simulink library "PowerFlowLib2013a"  (Simulink 8.1)
settings: Solver=ode45  StartTime=0.0  StopTime=10.0  RelTol=1e-3
undefined symbols (not defined in the file or in its folder): AirProp, C, F1, Fanmap, Fld1, Fld2, fueltankdata, HydProp, HydraulicLoad, IBFD_exc, L, LoadFluidProps, magnitude, MSSN, n_alghts, PumpProp, pwr_alghts, R_fd_exc, Rcore, Ts, VBFD_exc
libraries: PowerFlowLib x32, simulink x14, powerlib_extras x2, dspstat3 x2
(part 1 of 11)
settings Model: Creator=mwillms4  LastModifiedBy=srikanthan

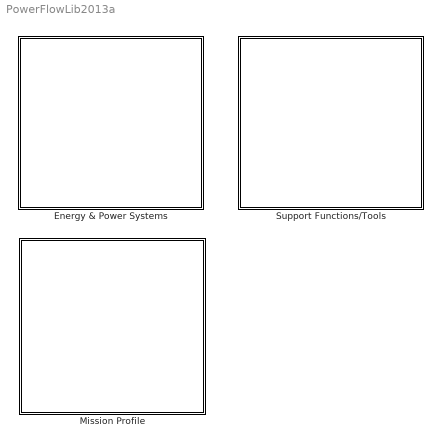
== system PowerFlowLib2013a ==
  Energy & Power Systems : Subsystem
      mask Display: color('white')
  Mission Profile : Subsystem
      mask Display: color('white')
  Support Functions/Tools : Subsystem
      mask Display: color('white')

== system PowerFlowLib2013a/Energy & Power Systems ==
  Additional Systems : Subsystem
  Electrical : Subsystem
  Hydraulic : Subsystem
  Thermal : Subsystem

== system PowerFlowLib2013a/Mission Profile ==
  Mission Profile : Subsystem  mask(MISSION PROFILE SELECT){mssn_check=off, mssn_prof=MSSN, del_P=0, del_T=0, del_rho=0, pres_msl=101.3, temp_msl=15, dens_msl=1.229}
      mask prompts: mssn_check "Define new mission?"; mssn_prof "Mission Profile Variable (from workspace)"; del_P "Pres. deviation from standard atmospheric conditions [kPa]"; del_T "Temp. deviation from standard atmospheric conditions [°C]"; del_rho "Density Deviation from standard"; pres_msl "MSL Pressure [kPa]"; temp_msl "MSL Temperature [°C]"; dens_msl "MSL Density [kg/m³]"
      mask help:
      | Select the MATLAB workspace variable that contains mission specifications. This variable should be created with the automated code included with the PowerFlow toolset.
      |
      | Also specify deviations from standard atmospheric conditions.
      mask init:
      | %{
      | h      = get_param(gcb,'handle');   % Get block handle
      | blk    = gcb; 
      | hblock = get(h);     % Parse out handles structure 
      | 
      | % altitude - row 2 of mission profile
      | set_param([blk,'/ALT'],'Table',[hblock.mssn_prof,'(2,:)'])
      | % mach number - row 22 of mission profile
      | set_param([blk,'/MACH'],'Table',[hblock.mssn_prof,'(22,:)'])
      | % mission phase - row 21 of mission profile
      | set_param([blk,'/MSSN Phase'],'Table',[hblock.mssn_prof,'(21,:)'])
      | % engine 1 on/off - row 6 of mission profile
      | set_param([blk,'/Engine 1'],'Table',[hblock.mssn_prof,'(6,:)'])
      | % engine 2 on/off - row 10 of mission profile
      | set_param([blk,'/Engine 2'],'Table',[hblock.mssn_prof,'(10,:)'])
      | % APU on/off - row 3 of mission profile
      | set_param([blk,'/APU'],'Table',[hblock.mssn_prof,'(3,:)'])
      | % taxi lights - row 16 of mission profile
      | set_param([blk,'/Taxi Lights'],'Table',[hblock.mssn_prof,'(16,:)'])
      | % landing lights - row 17 of mission profile
      | set_param([blk,'/Landing Lights'],'Table',[hblock.mssn_prof,'(17,:)'])
      | % pressurization - row 20 of mission profile
      | set_param([blk,'/Pressurization'],'Table',[hblock.mssn_prof,'(20,:)'])
      | % flaps - row 19 of mission profile
      | set_param([blk,'/Flaps'],'Table',[hblock.mssn_prof,'(19,:)'])
      | 
      | clear h blk hblock
      | %}
      mask Callback mssn_check:
      | h      = get_param(gcb,'handle');   % Get block handle
      | blk    = gcb;
      | hblock = get(h);     % Parse out handles structure
      | 
      | if strcmp(hblock.mssn_check,'on') == 1;
      |     % call mission profile creator file
      |     MSSNMain;
      |     % bring command window to focus
      |     commandwindow;
      | 
      |     set_param(gcb,'mssn_check','off')
      | end
      | clear h hblock blk
      mask Callback mssn_prof:
      | h      = get_param(gcb,'handle');   % Get block handle
      | blk    = gcb;
      | hblock = get(h);     % Parse out handles structure
      | 
      | if ((exist(hblock.mssn_prof) == 0) && (strcmp('blank',hblock.mssn_prof) ~= 1))
      |     error('Error in field "Mission Profile Variable (from workspace)".  Variable does not exist in workspace.');
      | end
      | 
      | clear h blk hblock
